simulink model "test_vrml"  (R2019a)
settings: Solver=VariableStepAuto  StartTime=0.0  StopTime=10.0  RelTol=1e-3
libraries: blocklib x1, vrlib x1
settings Model: Creator=Imanol  LastModifiedBy=Imanol

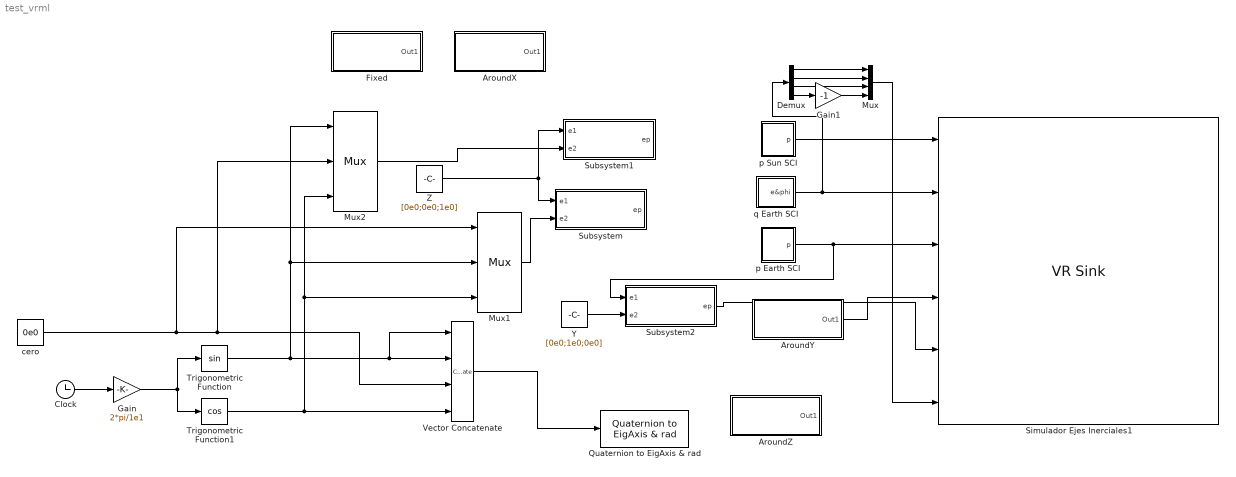
== system test_vrml ==
  AroundX : Subsystem
  AroundY : Subsystem
  AroundZ : Subsystem
  Clock : Clock
  Demux : Demux
  Fixed : Subsystem
  Gain : Gain  Gain=2*pi/1e1
  Gain1 : Gain  Gain=-1
  Mux : Mux
  Mux1 : Mux  Inputs=3
  Mux2 : Mux  Inputs=3
  Quaternion to EigAxis & rad : blocklib/Quaternion to EigAxis & rad  SystemSampleTime=-1
      settings: SourceProductName=Custom Library
  Simulador Ejes Inerciales1 : vrlib/VR Sink  InstantiateOnLoad=on  SampleTime=1e-2  ViewEnable=on  RemoteChange=off  RemoteView=off  FieldsWritten=StarSun.translation.3.1.1.double#PlanetEarth.rotation.4.1.1.double#PlanetEarth.translation.3.1.1.double#BillSun.rotation.4.1.1.double#BillEarth.rotation.4.1.1.double#BodyCoor.rotation.4.1.1.double  WorldFileName=myworldV4.wrl  AutoView=off  VideoDimensions=[]  AllowVariableSize=off
      settings: SourceProductBaseCode=VR
  Subsystem : Subsystem
  Subsystem1 : Subsystem
  Subsystem2 : Subsystem
  Trigonometric Function : Trigonometry
  Trigonometric Function1 : Trigonometry  Operator=cos
  Vector Concatenate : Concatenate  NumInputs=4
  Y : Constant  Value=[0e0;1e0;0e0]
  Z : Constant  Value=[0e0;0e0;1e0]
  cero : Constant  Value=0e0
  p Earth SCI : Subsystem
  p Sun SCI : Subsystem
  q Earth SCI : Subsystem
  wires:
  Clock/1 -> Gain/1
  Gain/1 -> Trigonometric Function1/1, Trigonometric Function/1
  Trigonometric Function1/1 -> Mux2/3, Mux1/3, Vector Concatenate/4
  cero/1 -> Vector Concatenate/3, Mux2/2, Mux1/1
  Vector Concatenate/1 -> Quaternion to EigAxis & rad/1
  Trigonometric Function/1 -> Vector Concatenate/2, Vector Concatenate/1, Mux2/1, Mux1/2
  Z/1 -> Subsystem/1(e1), Subsystem1/1(e1)
  Mux2/1 -> Subsystem1/2(e2)
  Mux1/1 -> Subsystem/2(e2)
  q Earth SCI/1(e&phi) -> Demux/1, Simulador Ejes Inerciales1/2
  p Earth SCI/1(p) -> Subsystem2/1(e1), Simulador Ejes Inerciales1/3
  p Sun SCI/1(p) -> Simulador Ejes Inerciales1/1
  Demux/1 -> Mux/1
  Demux/2 -> Mux/2
  Demux/3 -> Mux/3
  Demux/4 -> Gain1/1
  Gain1/1 -> Mux/4
  Mux/1 -> Simulador Ejes Inerciales1/6
  AroundY/1(Out1) -> Simulador Ejes Inerciales1/4
  Y/1 -> Subsystem2/2(e2)
  Subsystem2/1(ep) -> Simulador Ejes Inerciales1/5

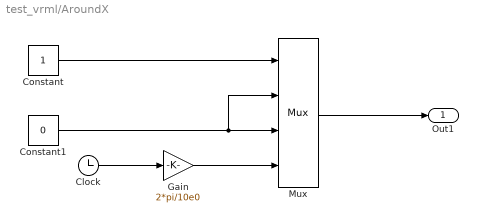
== system test_vrml/AroundX ==
  Clock : Clock
  Constant : Constant
  Constant1 : Constant  Value=0
  Gain : Gain  Gain=2*pi/10e0
  Mux : Mux
  Out1 : Outport
  wires:
  Clock/1 -> Gain/1
  Mux/1 -> Out1/1
  Gain/1 -> Mux/4
  Constant1/1 -> Mux/2, Mux/3
  Constant/1 -> Mux/1

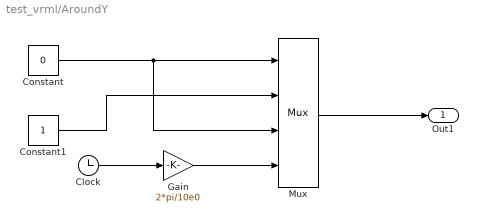
== system test_vrml/AroundY ==
  Clock : Clock
  Constant : Constant  Value=0
  Constant1 : Constant
  Gain : Gain  Gain=2*pi/10e0
  Mux : Mux
  Out1 : Outport
  wires:
  Clock/1 -> Gain/1
  Mux/1 -> Out1/1
  Gain/1 -> Mux/4
  Constant/1 -> Mux/3, Mux/1
  Constant1/1 -> Mux/2

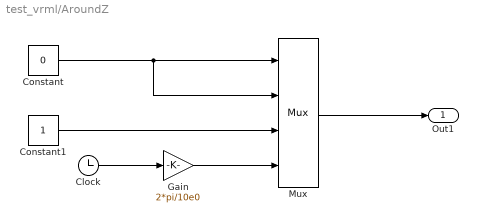
== system test_vrml/AroundZ ==
  Clock : Clock
  Constant : Constant  Value=0
  Constant1 : Constant
  Gain : Gain  Gain=2*pi/10e0
  Mux : Mux
  Out1 : Outport
  wires:
  Clock/1 -> Gain/1
  Mux/1 -> Out1/1
  Gain/1 -> Mux/4
  Constant1/1 -> Mux/3
  Constant/1 -> Mux/2, Mux/1

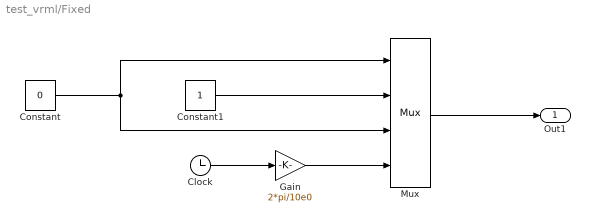
== system test_vrml/Fixed ==
  Clock : Clock
  Constant : Constant  Value=0
  Constant1 : Constant
  Gain : Gain  Gain=2*pi/10e0
  Mux : Mux
  Out1 : Outport
  wires:
  Clock/1 -> Gain/1
  Mux/1 -> Out1/1
  Gain/1 -> Mux/4
  Constant1/1 -> Mux/2
  Constant/1 -> Mux/3, Mux/1

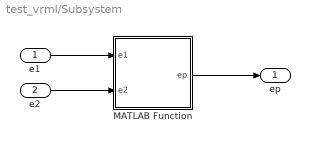
== system test_vrml/Subsystem ==
  e1 : Inport
  e2 : Inport  Port=2
  MATLAB Function : MATLAB Function  TreatAsAtomicUnit=on
  ep : Outport
  wires:
  e1/1 -> MATLAB Function/1(e1)
  e2/1 -> MATLAB Function/2(e2)
  MATLAB Function/1(ep) -> ep/1

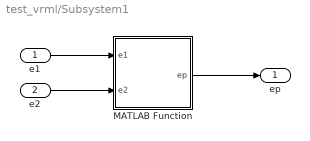
== system test_vrml/Subsystem1 ==
  e1 : Inport
  e2 : Inport  Port=2
  MATLAB Function : MATLAB Function  TreatAsAtomicUnit=on
  ep : Outport
  wires:
  e1/1 -> MATLAB Function/1(e1)
  e2/1 -> MATLAB Function/2(e2)
  MATLAB Function/1(ep) -> ep/1

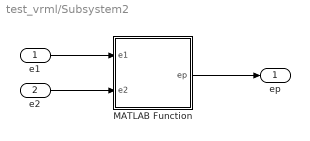
== system test_vrml/Subsystem2 ==
  e1 : Inport
  e2 : Inport  Port=2
  MATLAB Function : MATLAB Function  TreatAsAtomicUnit=on
  ep : Outport
  wires:
  e1/1 -> MATLAB Function/1(e1)
  e2/1 -> MATLAB Function/2(e2)
  MATLAB Function/1(ep) -> ep/1

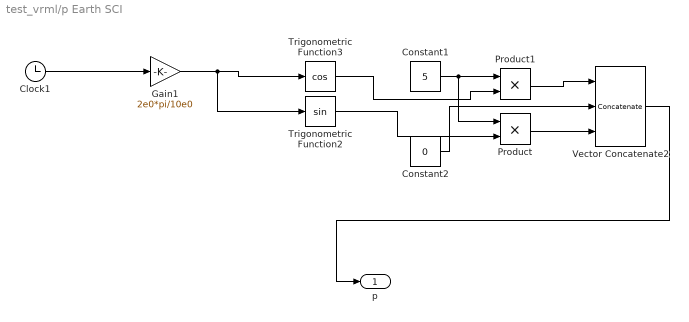
== system test_vrml/p Earth SCI ==
  Clock1 : Clock
  Constant1 : Constant  Value=5
  Constant2 : Constant  Value=0
  Gain1 : Gain  Gain=2e0*pi/10e0
  Product : Product
  Product1 : Product
  Trigonometric Function2 : Trigonometry
  Trigonometric Function3 : Trigonometry  Operator=cos
  Vector Concatenate2 : Concatenate  NumInputs=3
  p : Outport
  wires:
  Constant1/1 -> Product/1, Product1/1
  Trigonometric Function3/1 -> Product1/2
  Product/1 -> Vector Concatenate2/3
  Trigonometric Function2/1 -> Product/2
  Product1/1 -> Vector Concatenate2/1
  Constant2/1 -> Vector Concatenate2/2
  Clock1/1 -> Gain1/1
  Gain1/1 -> Trigonometric Function2/1, Trigonometric Function3/1
  Vector Concatenate2/1 -> p/1

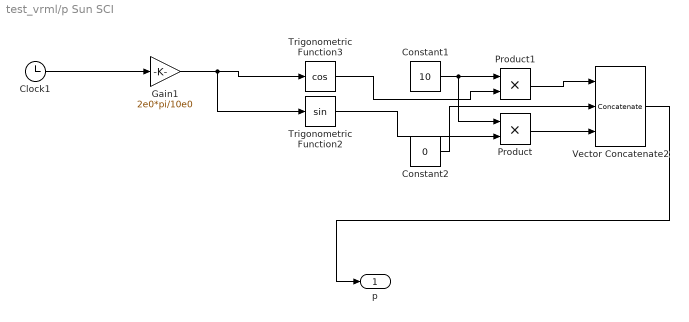
== system test_vrml/p Sun SCI ==
  Clock1 : Clock
  Constant1 : Constant  Value=10
  Constant2 : Constant  Value=0
  Gain1 : Gain  Gain=2e0*pi/10e0
  Product : Product
  Product1 : Product
  Trigonometric Function2 : Trigonometry
  Trigonometric Function3 : Trigonometry  Operator=cos
  Vector Concatenate2 : Concatenate  NumInputs=3
  p : Outport
  wires:
  Constant1/1 -> Product/1, Product1/1
  Trigonometric Function3/1 -> Product1/2
  Product/1 -> Vector Concatenate2/3
  Trigonometric Function2/1 -> Product/2
  Product1/1 -> Vector Concatenate2/1
  Constant2/1 -> Vector Concatenate2/2
  Clock1/1 -> Gain1/1
  Gain1/1 -> Trigonometric Function2/1, Trigonometric Function3/1
  Vector Concatenate2/1 -> p/1

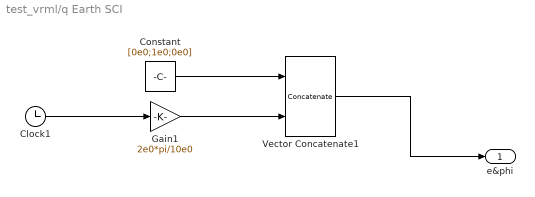
== system test_vrml/q Earth SCI ==
  Clock1 : Clock
  Constant : Constant  Value=[0e0;1e0;0e0]
  Gain1 : Gain  Gain=2e0*pi/10e0
  Vector Concatenate1 : Concatenate
  e&phi : Outport
  wires:
  Constant/1 -> Vector Concatenate1/1
  Clock1/1 -> Gain1/1
  Gain1/1 -> Vector Concatenate1/2
  Vector Concatenate1/1 -> e&phi/1

== matlab function test_vrml/Subsystem1/MATLAB Function ==
  data: e1 input; ep output; e2 input
function ep = fcn(e1, e2)
e = cross(e1, e2);
e = e / norm(e);
phi = acos(dot(e1, e2) / norm(e1) * norm(e2));
ep = [e(2); e(1); e(3); phi];

== matlab function test_vrml/Subsystem/MATLAB Function ==
  data: e1 input; ep output; e2 input
function ep = fcn(e1, e2)
e = cross(e1, e2);
e = e / norm(e);
phi = acos(dot(e1, e2) / norm(e1) * norm(e2));
ep = [e(2); e(1); e(3); phi];

== matlab function test_vrml/Subsystem2/MATLAB Function ==
  data: e1 input; ep output; e2 input
function ep = fcn(e1, e2)
e = cross(e1, e2);
e = e / norm(e);
phi = acos(dot(e1, e2) / norm(e1) * norm(e2));
ep = [e(1); e(2); e(3); phi];
